simulink model "mod_torque_bloque"  (R2023b)
settings: Solver=VariableStepAuto  StartTime=0.0  StopTime=10.0  RelTol=1e-3
values from neighbouring files (symbols this model uses):
  b_eq = b_eq_max    (= 2.40277777778e-05)    [analisis_estabilidad.m]    (also in parametros.m = 2.19444444444e-05; parametros_sim.m = 2.19444444444e-05)
  k_l = (m*l_cm + m_l*l_l)*g    (= 2.4516625)    [analisis_estabilidad.m]    (also in parametros.m = 0.25; parametros_sim.m)
  L_d = 6.6    [analisis_estabilidad.m]    (also in parametros.m = 0.0066; parametros_sim.m; polosyceros.m = L_d^3)
  L_ls = 0.8    [analisis_estabilidad.m]    (also in parametros.m = 0.0008; parametros_sim.m)
  L_q = 5.8    [analisis_estabilidad.m]    (also in parametros.m = 0.0058; parametros_sim.m; polosyceros.m = L_q^3)
  lambda_m = 0.016    [analisis_estabilidad.m]    (also in parametros.m; parametros_sim.m)
  P_p = 3    [analisis_estabilidad.m]    (also in parametros.m; parametros_sim.m)
  r = 120    [analisis_estabilidad.m]    (also in parametros.m; parametros_sim.m)
settings Model: Creator=Marti  LastModifiedBy=Marti

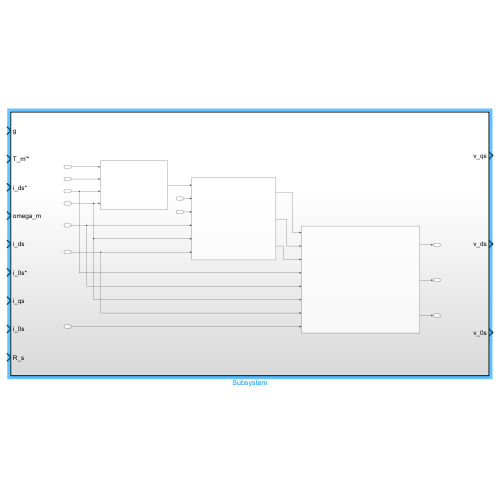
[thumbnail: Simulink's stored preview of the top-level diagram]
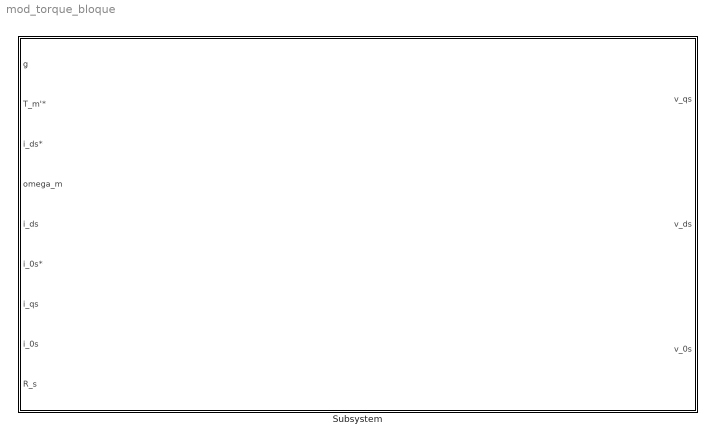
== system mod_torque_bloque ==
  Subsystem : Subsystem

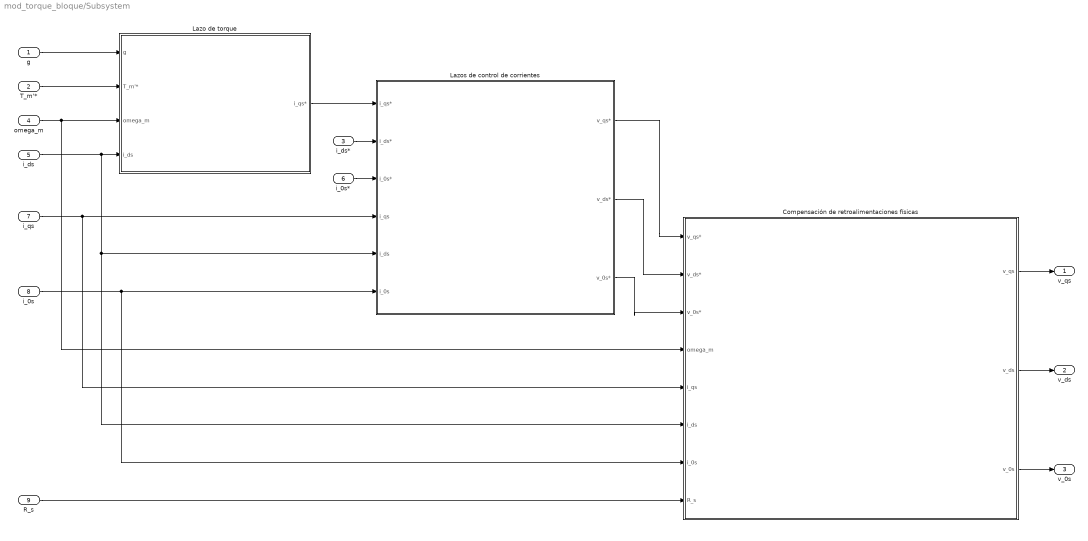
== system mod_torque_bloque/Subsystem ==
  g : Inport
  T_m'* : Inport  Port=2
  i_ds* : Inport  Port=3
  omega_m : Inport  Port=4
  i_ds : Inport  Port=5
  i_0s* : Inport  Port=6
  i_qs : Inport  Port=7
  i_0s : Inport  Port=8
  R_s : Inport  Port=9
  Compensación de retroalimentaciones físicas : Subsystem
  Lazo de torque : Subsystem
  Lazos de control de corrientes : Subsystem
  v_qs : Outport
  v_ds : Outport  Port=2
  v_0s : Outport  Port=3
  wires:
  Lazos de control de corrientes/3(v_0s*) -> Compensación de retroalimentaciones físicas/3(v_0s*)
  i_ds*/1 -> Lazos de control de corrientes/2(i_ds*)
  T_m'*/1 -> Lazo de torque/2(T_m'*)
  Lazos de control de corrientes/1(v_qs*) -> Compensación de retroalimentaciones físicas/1(v_qs*)
  Lazos de control de corrientes/2(v_ds*) -> Compensación de retroalimentaciones físicas/2(v_ds*)
  omega_m/1 -> Lazo de torque/3(omega_m), Compensación de retroalimentaciones físicas/4(omega_m)
  Lazo de torque/1(i_qs*) -> Lazos de control de corrientes/1(i_qs*)
  g/1 -> Lazo de torque/1(g)
  Compensación de retroalimentaciones físicas/3(v_0s) -> v_0s/1
  i_ds/1 -> Compensación de retroalimentaciones físicas/6(i_ds), Lazos de control de corrientes/5(i_ds), Lazo de torque/4(i_ds)
  Compensación de retroalimentaciones físicas/1(v_qs) -> v_qs/1
  i_0s*/1 -> Lazos de control de corrientes/3(i_0s*)
  Compensación de retroalimentaciones físicas/2(v_ds) -> v_ds/1
  i_qs/1 -> Compensación de retroalimentaciones físicas/5(i_qs), Lazos de control de corrientes/4(i_qs)
  i_0s/1 -> Compensación de retroalimentaciones físicas/7(i_0s), Lazos de control de corrientes/6(i_0s)
  R_s/1 -> Compensación de retroalimentaciones físicas/8(R_s)

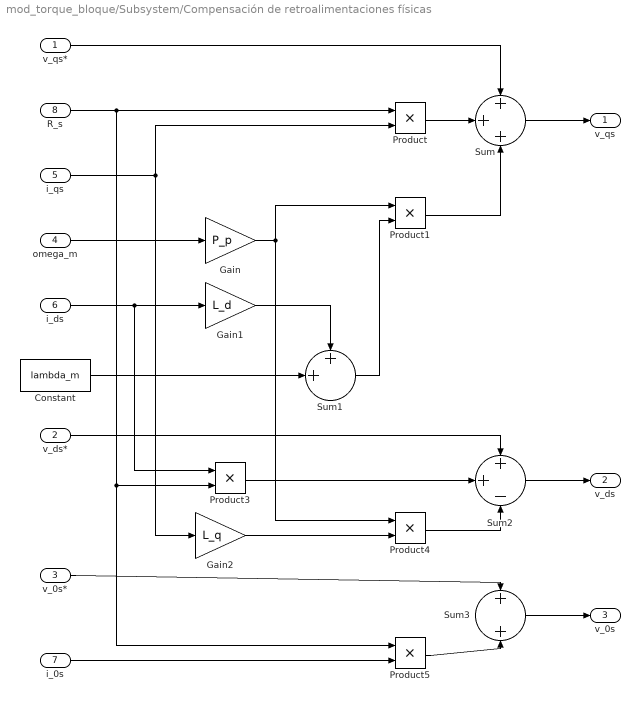
== system mod_torque_bloque/Subsystem/Compensación de retroalimentaciones físicas ==
  v_qs* : Inport
  v_ds* : Inport  Port=2
  v_0s* : Inport  Port=3
  omega_m : Inport  Port=4
  i_qs : Inport  Port=5
  i_ds : Inport  Port=6
  i_0s : Inport  Port=7
  R_s : Inport  Port=8
  Constant : Constant  Value=lambda_m
  Gain : Gain  Gain=P_p
  Gain1 : Gain  Gain=L_d
  Gain2 : Gain  Gain=L_q
  Product{,1,3..5} (5 alike) : Product
  Sum : Sum  Inputs=+++
  Sum1 : Sum  Inputs=++|
  Sum2 : Sum  Inputs=++-
  Sum3 : Sum
  v_qs : Outport
  v_ds : Outport  Port=2
  v_0s : Outport  Port=3
  wires:
  v_qs*/1 -> Sum/1
  R_s/1 -> Product5/1, Product3/2, Product/1
  i_qs/1 -> Gain2/1, Product/2
  Product/1 -> Sum/2
  Product1/1 -> Sum/3
  omega_m/1 -> Gain/1
  Gain/1 -> Product4/1, Product1/1
  Sum1/1 -> Product1/2
  Gain1/1 -> Sum1/1
  i_ds/1 -> Product3/1, Gain1/1
  Constant/1 -> Sum1/2
  v_ds*/1 -> Sum2/1
  Product3/1 -> Sum2/2
  Gain2/1 -> Product4/2
  Product4/1 -> Sum2/3
  v_0s*/1 -> Sum3/1
  Product5/1 -> Sum3/2
  i_0s/1 -> Product5/2
  Sum/1 -> v_qs/1
  Sum2/1 -> v_ds/1
  Sum3/1 -> v_0s/1

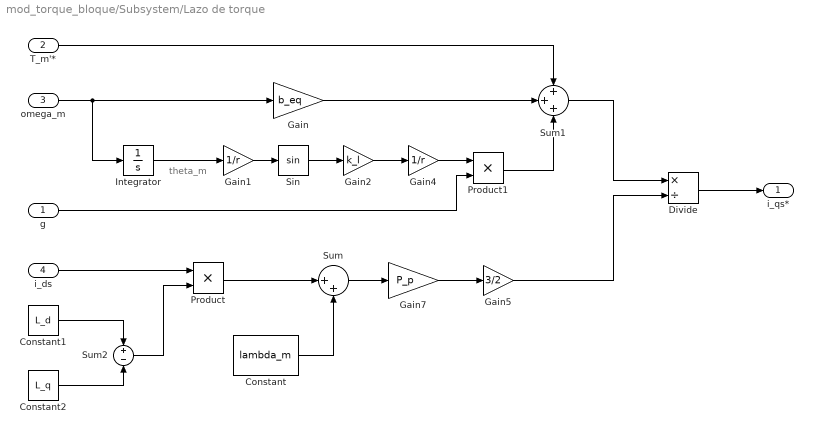
== system mod_torque_bloque/Subsystem/Lazo de torque ==
  note: theta_m
  g : Inport
  T_m'* : Inport  Port=2
  omega_m : Inport  Port=3
  i_ds : Inport  Port=4
  Constant : Constant  Value=lambda_m
  Constant1 : Constant  Value=L_d
  Constant2 : Constant  Value=L_q
  Divide : Product  Inputs=*/
  Gain : Gain  Gain=b_eq
  Gain1 : Gain  Gain=1/r
  Gain2 : Gain  Gain=k_l
  Gain4 : Gain  Gain=1/r
  Gain5 : Gain  Gain=3/2
  Gain7 : Gain  Gain=P_p
  Integrator : Integrator
  Product : Product
  Product1 : Product
  Sin : Trigonometry
  Sum : Sum  Inputs=|++
  Sum1 : Sum  Inputs=+++
  Sum2 : Sum  Inputs=+-
  i_qs* : Outport
  wires:
  omega_m/1 -> Gain/1, Integrator/1
  Gain/1 -> Sum1/2
  Integrator/1 -> Gain1/1
  Gain1/1 -> Sin/1
  Product1/1 -> Sum1/3
  Sum1/1 -> Divide/1
  T_m'*/1 -> Sum1/1
  Divide/1 -> i_qs*/1
  Sin/1 -> Gain2/1
  Gain2/1 -> Gain4/1
  Gain7/1 -> Gain5/1
  Gain5/1 -> Divide/2
  Gain4/1 -> Product1/1
  g/1 -> Product1/2
  Sum/1 -> Gain7/1
  Constant/1 -> Sum/2
  Constant2/1 -> Sum2/2
  Constant1/1 -> Sum2/1
  Sum2/1 -> Product/2
  i_ds/1 -> Product/1
  Product/1 -> Sum/1

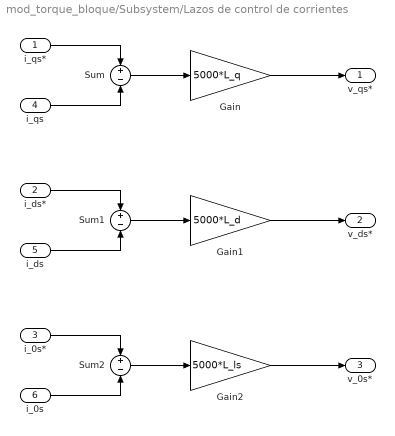
== system mod_torque_bloque/Subsystem/Lazos de control de corrientes ==
  i_qs* : Inport
  i_ds* : Inport  Port=2
  i_0s* : Inport  Port=3
  i_qs : Inport  Port=4
  i_ds : Inport  Port=5
  i_0s : Inport  Port=6
  Gain : Gain  Gain=5000*L_q
  Gain1 : Gain  Gain=5000*L_d
  Gain2 : Gain  Gain=5000*L_ls
  Sum : Sum  Inputs=+-
  Sum1 : Sum  Inputs=+-
  Sum2 : Sum  Inputs=+-
  v_qs* : Outport
  v_ds* : Outport  Port=2
  v_0s* : Outport  Port=3
  wires:
  i_ds*/1 -> Sum1/1
  i_ds/1 -> Sum1/2
  i_qs/1 -> Sum/2
  Gain/1 -> v_qs*/1
  Sum2/1 -> Gain2/1
  i_0s/1 -> Sum2/2
  i_0s*/1 -> Sum2/1
  Sum/1 -> Gain/1
  Gain2/1 -> v_0s*/1
  i_qs*/1 -> Sum/1
  Sum1/1 -> Gain1/1
  Gain1/1 -> v_ds*/1
